simulink model "Transmissionctrl"  (R2020a)
settings: Solver=VariableStepAuto  StartTime=0.0  StopTime=30  RelTol=1e-3
InitFcn:
  | Ne_vec=[799.9999999999999 1200 1600 2000 2400 2800 3200 3600 4000 4400 4800];
  | th_vec=[0;20;30;40;50;60;70;80;90;100];
  | EMAP=[-40 -44 -49 -53 -57 -61 -65 -70 -74 -78 -82;215 117 85 66 44 29 10 -2 -13 -22 -32;245 208 178 148 122 104 85 66 48 33 18;264 260 241 219 193 167 152 133 119 96 85;264 279 282 275 260 238 223 208 189 171 152;267 290 293 297 290 275 260 256 234 212 193;267 297 305 305 305 301 293 282 267 249 226;267 301 308 312 319 323 319 316 297 279 253;267 301 312 319 327 327 327 327 312 293 267;267 301 312 319 327 334 334 334 319 305 275];
undefined symbols (not defined in the file or in its folder): Converter_data, DOWN_TABLE, DOWN_TH_BP, Iei, sigbuilder_block, UP_TABLE, UP_TH_BP, Vehicle_data
settings Model: DataDictionary=Trans_ctrl.sldd  Creator=USER  LastModifiedBy=USER

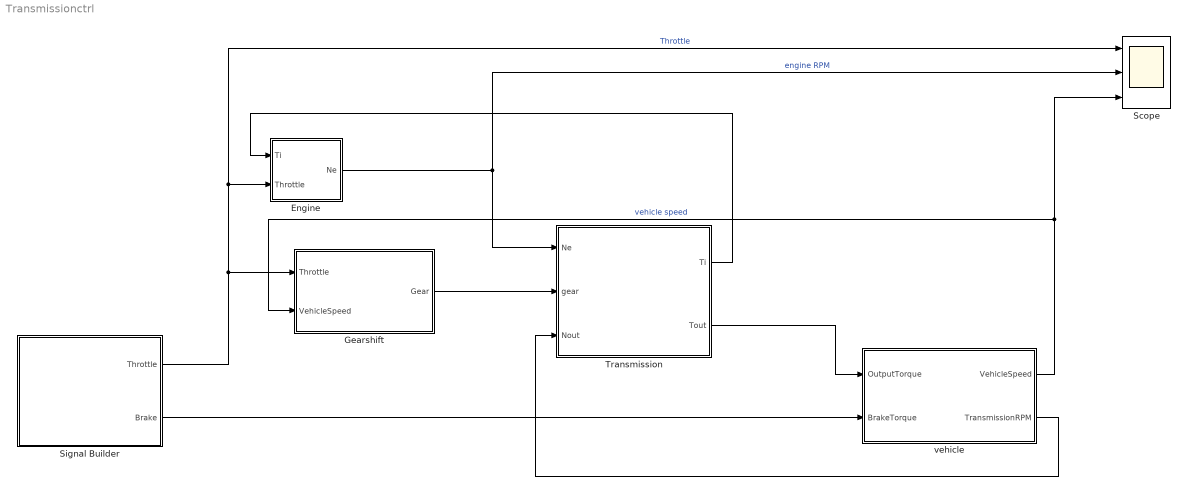
== system Transmissionctrl ==
  Engine : Subsystem
  Gearshift : Stateflow chart  TreatAsAtomicUnit=on
  Scope : Scope  NumInputPorts=3
  Signal Builder : Subsystem  Tag=STV Subsys  LoadFcn=sigbuilder_block('load');  StartFcn=sigbuilder_block('start');  StopFcn=sigbuilder_block('stop');  ClipboardFcn=sigbuilder_block('clipboard');  mask(Sigbuilder block){tuvar=[0:10]}
      mask help: Simulink:masks:SigbuilderBlock_MD
      mask init:
      | if ~strcmp(get_param(bdroot(gcbh),'SimulationStatus'),'stopped') tuvar = sigbuilder_block('maskInit'); end
      settings: CopyFcn=sigbuilder_block('copy');  DeleteFcn=sigbuilder_block('delete');  ModelCloseFcn=sigbuilder_block('modelClose');  PreSaveFcn=sigbuilder_block('preSave');  PauseFcn=sigbuilder_block('pause');  ContinueFcn=sigbuilder_block('continue');  NameChangeFcn=sigbuilder_block('namechange');  OpenFcn=sigbuilder_block('open',[6 30 1012.5 447.75 ]);  CloseFcn=sigbuilder_block('close');
      mask Display: plot(0, 0, 100, 100,[2, 2, 32, 32, 2], [68, 8, 8, 68, 68],[32, 2], [38, 38], [32, 19, 2],[53, 60, 44], [32, 17, 17, 2],[16, 16, 31, 31]);txt = getActiveGroup(gcbh);text(2, 100, txt,'verticalAlignment', 'top');
  Transmission : Subsystem
  vehicle : Subsystem  mask{Fdr=Vehicle_data(1), rload2=Vehicle_data(3), rload0=Vehicle_data(2), Rw=Vehicle_data(4), Iv=Vehicle_data(5), U=Vehicle_data(6)/Vehicle_data(4)*Vehicle_data(1)}
      mask prompts: Fdr "Final drive ratio"; rload2 "Aerodynamic drag"; rload0 "Drag friction at wheels"; Rw "wheel Radius"; Iv "Vehicle inertia"; U "Initial Transmission output speed"
  wires:
  Signal Builder/1(Throttle) -> Scope/1, Engine/2(Throttle), Gearshift/1(Throttle)  "Throttle"
  Engine/1(Ne) -> Scope/2, Transmission/1(Ne)  "engine RPM"
  Signal Builder/2(Brake) -> vehicle/2(BrakeTorque)
  Transmission/2(Tout) -> vehicle/1(OutputTorque)
  vehicle/2(TransmissionRPM) -> Transmission/3("\tNout")
  Transmission/1(Ti) -> Engine/1(Ti)
  vehicle/1(VehicleSpeed) -> Gearshift/2(VehicleSpeed), Scope/3  "vehicle speed"
  Gearshift/1(Gear) -> Transmission/2(gear)

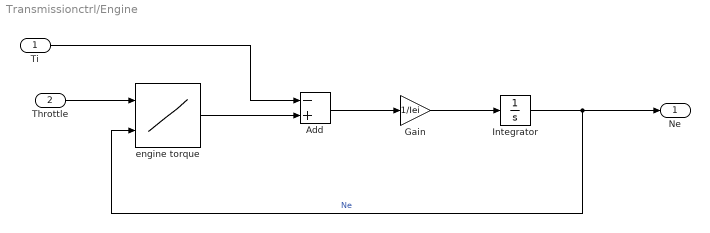
== system Transmissionctrl/Engine ==
  Ti : Inport
  Throttle : Inport  Port=2
  Add : Sum  Inputs=-+
  Gain : Gain  Gain=1/Iei
  Integrator : Integrator  InitialCondition=1000  LimitOutput=on  UpperSaturationLimit=6000  LowerSaturationLimit=600
  engine torque : Lookup_n-D  BreakpointsForDimension1=th_vec  BreakpointsForDimension2=Ne_vec  Table=EMAP  InternalRulePriority=Speed  RndMeth=Simplest  InputSameDT=on
  Ne : Outport
  wires:
  Ti/1 -> Add/1
  Add/1 -> Gain/1
  Integrator/1 -> Ne/1, engine torque/2  "Ne"
  Throttle/1 -> engine torque/1
  Gain/1 -> Integrator/1
  engine torque/1 -> Add/2

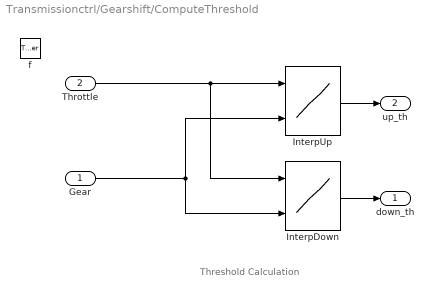
== system Transmissionctrl/Gearshift/ComputeThreshold ==
  note: Threshold Calculation
  Gear : Inport
  Throttle : Inport  Port=2
  f : TriggerPort  TriggerType=function-call  VariantControl=(inherit)
      settings: CopyFcn=Stateflow.SLINSF.SimulinkMan.removeBlockPreDeleteFcn  PreDeleteFcn=Stateflow.SLINSF.SimulinkMan.unsafePredeleteFcn
  InterpDown : Lookup_n-D  BreakpointsForDimension1=DOWN_TH_BP  BreakpointsForDimension2=[1:4]  Table=DOWN_TABLE  OutDataTypeStr=double  LockScale=on
  InterpUp : Lookup_n-D  BreakpointsForDimension1=UP_TH_BP  BreakpointsForDimension2=[1:4]  Table=UP_TABLE  OutDataTypeStr=double  LockScale=on
  down_th : Outport  InitialOutput=0  VectorParamsAs1DForOutWhenUnconnected=off
  up_th : Outport  Port=2  InitialOutput=0  VectorParamsAs1DForOutWhenUnconnected=off
  wires:
  InterpUp/1 -> up_th/1
  InterpDown/1 -> down_th/1
  Throttle/1 -> InterpDown/1, InterpUp/1
  Gear/1 -> InterpDown/2, InterpUp/2

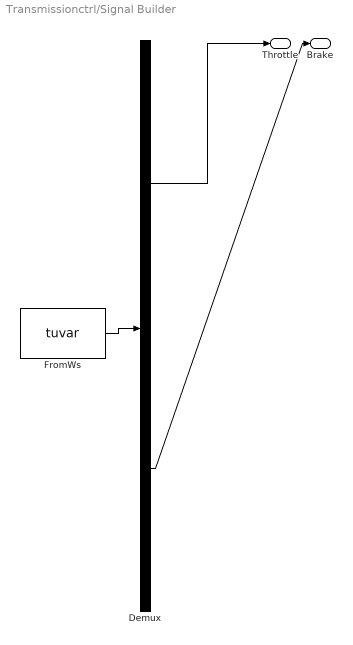
== system Transmissionctrl/Signal Builder ==
  Demux : Demux  Tag=STV Demux  Outputs=2
      settings: DisplayOption=none
  FromWs : FromWorkspace  Tag=STV FromWs  VariableName=tuvar
      SigBuilderData=|
      | common.afterFinalStr = 'Extrapolate'
      | common.sampleTime = 0
      | dataSet.timeRange = [0 50]
      | dataSet.name = 'Group 1'
      | sbobj.Groups.Name = 'Group 1'
      | sbobj.Groups.Signals(1).Name = 'Throttle'
      | sbobj.Groups.Signals(1).XData = [0 14.9 15 50]
      | sbobj.Groups.Signals(1).YData = [60 40 100 60]
      | sbobj.Groups.Signals(2).Name = 'Brake'
      | sbobj.Groups.Signals(2).XData = [0 25 50]
      | sbobj.Groups.Signals(2).YData = [0 0 0]
      | sbobj.Groups.TimeRange = [0 50]
  Throttle : Outport  Tag=STV Outport
  Brake : Outport  Tag=STV Outport  Port=2
  wires:
  Demux/1 -> Throttle/1
  FromWs/1 -> Demux/1
  Demux/2 -> Brake/1

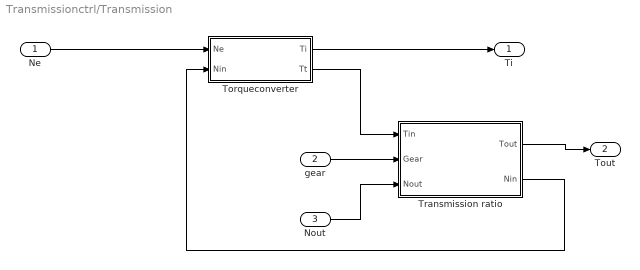
== system Transmissionctrl/Transmission ==
  Ne : Inport
  gear : Inport  Port=2
  "\tNout" : Inport  Port=3
  Torqueconverter : Subsystem  mask{Kfactor=Converter_data(:,2), speedratio=Converter_data(:,1), Torqueratio=Converter_data(:,3)}
      mask prompts: Kfactor "K factor"; speedratio "Speed Ratio"; Torqueratio "Torque Ratio"
  Transmission ratio : Subsystem
  Ti : Outport
  Tout : Outport  Port=2
  wires:
  Ne/1 -> Torqueconverter/1(Ne)
  Torqueconverter/1(Ti) -> Ti/1
  Torqueconverter/2(Tt) -> Transmission ratio/1(Tin)
  gear/1 -> Transmission ratio/2(Gear)
  "\tNout"/1 -> Transmission ratio/3(Nout)
  Transmission ratio/2(Nin) -> Torqueconverter/2(Nin)
  Transmission ratio/1(Tout) -> Tout/1

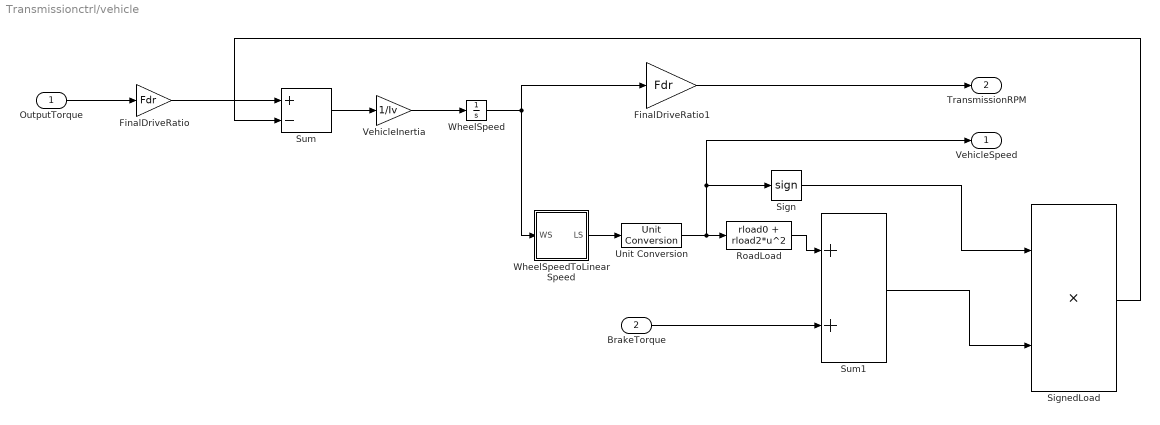
== system Transmissionctrl/vehicle ==
  OutputTorque : Inport  Unit=ft*lbf@torque
  BrakeTorque : Inport  Port=2  Unit=ft*lbf@torque
  FinalDriveRatio : Gain  Gain=Fdr  SaturateOnIntegerOverflow=on  OutDataTypeStr=Inherit: Same as input  ParamDataTypeStr=Inherit: Same as input
  FinalDriveRatio1 : Gain  Gain=Fdr  SaturateOnIntegerOverflow=on  OutDataTypeStr=Inherit: Same as input  ParamDataTypeStr=Inherit: Same as input
  RoadLoad : Fcn  Expr=rload0 + rload2*u^2
  Sign : Signum
  SignedLoad : Product  InputSameDT=on  SaturateOnIntegerOverflow=on  OutDataTypeStr=Inherit: Same as first input
  Sum : Sum  Inputs=+-  InputSameDT=on  SaturateOnIntegerOverflow=on  OutDataTypeStr=Inherit: Same as first input
  Sum1 : Sum  InputSameDT=on  SaturateOnIntegerOverflow=on  OutDataTypeStr=Inherit: Same as first input
  Unit Conversion : UnitConversion
  VehicleInertia : Gain  Gain=1/Iv  SaturateOnIntegerOverflow=on  OutDataTypeStr=Inherit: Same as input  ParamDataTypeStr=Inherit: Same as input
  WheelSpeed : Integrator  InitialCondition=U/Fdr  ZeroCross=off
  WheelSpeedToLinearSpeed : Subsystem
  VehicleSpeed : Outport  Unit=mph  VectorParamsAs1DForOutWhenUnconnected=off
  TransmissionRPM : Outport  Port=2  Unit=rpm  VectorParamsAs1DForOutWhenUnconnected=off
  wires:
  WheelSpeedToLinearSpeed/1(LS) -> Unit Conversion/1
  Unit Conversion/1 -> VehicleSpeed/1, Sign/1, RoadLoad/1
  FinalDriveRatio/1 -> Sum/1
  FinalDriveRatio1/1 -> TransmissionRPM/1
  WheelSpeed/1 -> WheelSpeedToLinearSpeed/1(WS), FinalDriveRatio1/1
  VehicleInertia/1 -> WheelSpeed/1
  OutputTorque/1 -> FinalDriveRatio/1
  Sum/1 -> VehicleInertia/1
  BrakeTorque/1 -> Sum1/2
  Sum1/1 -> SignedLoad/2
  SignedLoad/1 -> Sum/2
  RoadLoad/1 -> Sum1/1
  Sign/1 -> SignedLoad/1

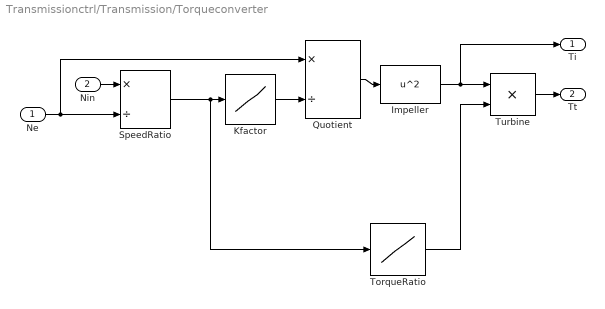
== system Transmissionctrl/Transmission/Torqueconverter ==
  Ne : Inport
  Nin : Inport  Port=2
  Impeller : Fcn  Expr=u^2
  Kfactor : Lookup_n-D  NumberOfTableDimensions=1  BreakpointsForDimension1=speedratio  Table=Kfactor  SaturateOnIntegerOverflow=on  InputSameDT=on
  Quotient : Product  Inputs=*/  InputSameDT=on  SaturateOnIntegerOverflow=on  OutDataTypeStr=Inherit: Same as first input
  SpeedRatio : Product  Inputs=*/  InputSameDT=on  SaturateOnIntegerOverflow=on  OutDataTypeStr=Inherit: Same as first input
  TorqueRatio : Lookup_n-D  NumberOfTableDimensions=1  BreakpointsForDimension1=speedratio  Table=Torqueratio  SaturateOnIntegerOverflow=on  InputSameDT=on
  Turbine : Product  InputSameDT=on  SaturateOnIntegerOverflow=on  OutDataTypeStr=Inherit: Same as first input
  Ti : Outport  VectorParamsAs1DForOutWhenUnconnected=off
  Tt : Outport  Port=2  VectorParamsAs1DForOutWhenUnconnected=off
  wires:
  Turbine/1 -> Tt/1
  Nin/1 -> SpeedRatio/1
  Ne/1 -> SpeedRatio/2, Quotient/1
  SpeedRatio/1 -> TorqueRatio/1, Kfactor/1
  Impeller/1 -> Turbine/1, Ti/1
  Kfactor/1 -> Quotient/2
  Quotient/1 -> Impeller/1
  TorqueRatio/1 -> Turbine/2

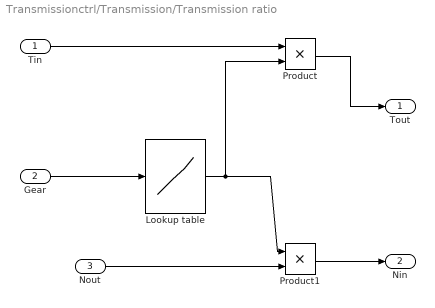
== system Transmissionctrl/Transmission/Transmission ratio ==
  Tin : Inport  Unit=ft*lbf@torque
  Gear : Inport  Port=2  Unit=1
  Nout : Inport  Port=3  Unit=rpm
  Lookup table : Lookup_n-D  NumberOfTableDimensions=1  BreakpointsForDimension1=[1 2 3 4]  Table=[2.393 1.450 1.000 0.677]  ExtrapMethod=Clip  OutDataTypeStr=double  SaturateOnIntegerOverflow=on  InputSameDT=on  LockScale=on
  Product : Product  InputSameDT=on  SaturateOnIntegerOverflow=on  OutDataTypeStr=Inherit: Same as first input
  Product1 : Product  InputSameDT=on  SaturateOnIntegerOverflow=on  OutDataTypeStr=Inherit: Same as first input
  Tout : Outport  Unit=ft*lbf@torque  VectorParamsAs1DForOutWhenUnconnected=off
  Nin : Outport  Port=2  Unit=rpm  VectorParamsAs1DForOutWhenUnconnected=off
  wires:
  Tin/1 -> Product/1
  Lookup table/1 -> Product1/1, Product/2
  Gear/1 -> Lookup table/1
  Nout/1 -> Product1/2
  Product1/1 -> Nin/1
  Product/1 -> Tout/1

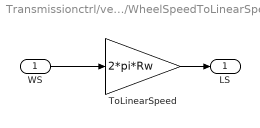
== system Transmissionctrl/vehicle/WheelSpeedToLinearSpeed ==
  WS : Inport  Unit=rpm
  ToLinearSpeed : Gain  Gain=2*pi*Rw  SaturateOnIntegerOverflow=on  OutDataTypeStr=Inherit: Same as input  ParamDataTypeStr=Inherit: Same as input
  LS : Outport  Unit=ft/min  VectorParamsAs1DForOutWhenUnconnected=off
  wires:
  ToLinearSpeed/1 -> LS/1
  WS/1 -> ToLinearSpeed/1

== stateflow chart Transmissionctrl/Gearshift ==
  settings: updateMethod=DISCRETE  sampleTime=0.04
  state selection_state [parallel]
    during:
    [down_th, up_th] = ComputeThreshold(Gear,Throttle);
    settings: executionOrder=2
    state steady_state
    state upshifting
    state downshifting
    (default) -> steady_state
    steady_state -> upshifting [order 1] : [VehicleSpeed > up_th]
    steady_state -> downshifting [order 2] : [VehicleSpeed < down_th]
    downshifting -> steady_state [order 2] : [VehicleSpeed > down_th]
    downshifting -> steady_state [order 1] : after(TWAIT,tick)
        | [VehicleSpeed <= down_th]
        | {gear_state.DOWN}
    upshifting -> steady_state [order 1] : after(TWAIT,tick)
        | [VehicleSpeed >= up_th]
        | {gear_state.UP}
    upshifting -> steady_state [order 2] : [VehicleSpeed < up_th]
  state gear_state [parallel]
    settings: executionOrder=1
    state first
      entry:
      Gear = 1;
    state second
      entry:
      Gear = 2;
    state third
      entry:
      Gear = 3;
    state fourth
      entry:
      Gear = 4;
    (default) -> first
    second -> third [order 1] : UP
    first -> second : UP
    third -> fourth [order 1] : UP
    third -> second [order 2] : DOWN
    second -> first [order 2] : DOWN
    fourth -> third : DOWN
  state [down_th,up_th] = ComputeThreshold(Gear,Throttle) [function]
  data: Gear function_input; Throttle function_input; down_th function_output; up_th function_output; Throttle input double; VehicleSpeed input double; Gear output fixdt(0,8,5) [1..4]; TWAIT parameter fixdt(0,8,6); down_th local double; up_th local double
  events: DOWN local EITHER_EDGE_EVENT; UP local EITHER_EDGE_EVENT
